simulink model "UNCCModel"  (R2018b)
settings: Solver=ode4  StartTime=0.0  StopTime=Inf  FixedStep=0.025  RelTol=1e-3  EnableMultiTasking=on
PreLoadFcn:
  | preLoadCallback
StartFcn:
  | startCallback
StopFcn:
  | stopCallback
model workspace (MAT data in the model file):
  Ts = 0.025
undefined symbols (not defined in the file or in its folder): acA2000, Ace, Basler, Freerun_FIX_YAW, PoCL
libraries: slrtlib x3, xpcbitflowlib x3, xpcvideoutillib x2, xpcobsoletelib x1, xpcrtudplib x1
(part 2 of 3)

== matlab function UNCCModel/cam3B/Dot_detector_pitch ==
  data: uOut output; u input; roiDims input; locationMethod input; dotConfig input; centroidOverrideCommand input; rCentroidManualOverride input; clusteringParameters input; rCentroidAuto input; r1Img output; r2Img output; rCentroidImg output; viewOptions input
function [uOut,r1Img,r2Img,rCentroidImg] =...
    dotFinder(u,roiDims, locationMethod, dotConfig,centroidOverrideCommand,rCentroidManualOverride,clusteringParameters,rCentroidAuto,viewOptions)
%#codegen
% EXPLANATION OF INPUTS
% u = source image
% roiDims = 4 by 1 vector containing ROI dimensions
% locationMethod = 0 for centroid based dot location
% locationMethod = 1 for cluster based dot location (longer runtime but
% more robust
% dotConfig = 0 for horizontally arranged dots
% dotConfig = 1 for vertically arranged dots
% centroidOverrideCommand = 0 for automatic movemennt of ROI
% centroidOverrideCommand = 1 to use user input as ROI location
% rCentroidManualOverride: 2 element vector where element 1 is x or column
% of ROI centroid and element 2 is y or row of ROI, both of which are
% manually enetered by used
% rCentroidAuto: 2 element vector where element 1 is x or column of ROI
% centroid and element 2 is y or row of ROI, both of which are
% automatically generated from previous iteration
% viewOptions : 8 element vector where each element is a binary on/off
% switch to a certain part of the output view window
%
% WHAT THIS CODE IS
% Method : Centroid Only
% 
% This code is a first attempt at rewriting the code to allow for adaptable
% implemmentation.
% Adaptable implemmentation will ultimately include:
% switch to change between DB clustering and centroid method
% 



%%%%%%%%%%%%%%%%%%%%
% SET ROI DIMENSIONS
%%%%%%%%%%%%%%%%%%%%
[ roiHalfwidth, roiHalfheight ] = getROIDimensions(setToBinary(dotConfig),roiDims); 

%%%%%%%%%%%%%%%%%%%%
% PARSE INPUTS
%%%%%%%%%%%%%%%%%%%%

[dotConfig, locationMethod, centroidOverrideCommand ,rCentroidManualOverride ,viewOptions,roiHalfwidth, roiHalfheight]...
    =parseInputs(dotConfig, locationMethod, centroidOverrideCommand ,rCentroidManualOverride ,viewOptions,roiHalfwidth, roiHalfheight);

%%%%%%%%%%%%%%%%%%%%
%%SET ROI LOCATION%%
%%%%%%%%%%%%%%%%%%%%
rCentroid = rCentroidAuto;
if centroidOverrideCommand == 1  %Override with user input if commanded to do so
    rCentroid = rCentroidManualOverride;
end

%%%%%%%%%%%%%%%%%%%%%%%%%%%%%%%%%%%%
% EXTRACT ROI FROM ORIGIONAL IMAGE %
%%%%%%%%%%%%%%%%%%%%%%%%%%%%%%%%%%%%
roi=u(rCentroid(2) - roiHalfheight : rCentroid(2) + roiHalfheight , rCentroid(1) - roiHalfwidth : rCentroid(1) + roiHalfwidth);

%%%%%%%%%%%%%%%%%%%%%%%%%%%%%
%%%%OTSUS METHOD THRESHOLDING
%%%%%%%%%%%%%%%%%%%%%%%%%%%%%
roi=threshold(roi);


%%%%%%%%%%%%%%%%
% DOT LOCATION %
%%%%%%%%%%%%%%%%
%Preallocate to avoid "Variable undefined on some iteration paths" compile
%error
r1ROI        = [0,0]; r2ROI        = [0,0]; rCentroidROI = [0,0];
if locationMethod == 0; %USE CENTROID BASED METHOD
    if dotConfig == 0 %%HORIZONTAL DOTS
        [r1ROI,r2ROI,rCentroidROI] = centroidMethodHorizontal(roi,roiHalfwidth,roiHalfheight);
    else                %%VERTICAL DOTS
        [r1ROI,r2ROI,rCentroidROI] = centroidMethodVertical(roi,roiHalfwidth,roiHalfheight);
    end
else %USE CLUSTERING BASED METHOD (NOT CURRENTLY IMPLEMENTED)
    %%%REPLACE THIS CODE WITH CLUSTERING METHOD WHEN IMPLEMENTING
    %%%UNCOMMENT CODE BELOW ONCE clusterMethod FUNCTION IS WRITTEN
    %%%[r1ROI,r2ROI,rCentroidROI] = clusterMethod(roi,clusteringParameters);
    if dotConfig == 0 %%HORIZONTAL DOTS
        [r1ROI,r2ROI,rCentroidROI] = centroidMethodHorizontal(roi,roiHalfwidth,roiHalfheight);
    else                %%VERTICAL DOTS
        [r1ROI,r2ROI,rCentroidROI] = centroidMethodVertical(roi,roiHalfwidth,roiHalfheight);
    end
end
%%%%%%%%%%%%%%%%%%%%%%%%%
%%%%PARSE DOT LOCATIONS %
%%%%%%%%%%%%%%%%%%%%%%%%%
%IF DOT CENTER LOCATION ALGORITHM HAS FAILED (OUTPUT = NONSENSE) THEN
%OVERRIDE CENTROID COORDINATES WITH DEFAULT VALUES TO PREVENT PROBLEMS
%LATER
[r1ROI,r2ROI,rCentroidROI] = parseDotLocations(dotConfig,r1ROI,r2ROI,rCentroidROI,roiHalfwidth,roiHalfheight);

%%%%%%%%%%%%%%%%%%%%%%%%%%%%%%%%%%%%%%%%%%%%%%%%%%%
%%%%TRANSFORM BACK TO ORIGIONAL IMAGE COORDINATES %
%%%%%%%%%%%%%%%%%%%%%%%%%%%%%%%%%%%%%%%%%%%%%%%%%%%
%Preallocate to avoid "Variable undefined on some iteration paths" compile
%error
r1Img         = [0,0]; r2Img         = [0,0]; rCenntroidImg = [0,0];

if dotConfig == 0  %HORIZONTALLY ARRANGED DOTS
    [r1Img, r2Img, rCentroidImg] = convertCoordinatesHorizontal(r1ROI,r2ROI,rCentroid,roiHalfwidth,roiHalfheight);
else % VERTICALLY ARRANGED DOTS
    [r1Img, r2Img, rCentroidImg] = convertCoordinatesVertical(r1ROI,r2ROI,rCentroid,roiHalfwidth,roiHalfheight);
end
%%%%%%%%%%%%%%%%%%%%%
% DRAW OUTPUT IMAGE %
%%%%%%%%%%%%%%%%%%%%%

uOut  =  drawOutputImage(viewOptions,u,roi,r1Img,r2Img,rCentroid,r1ROI,r2ROI,roiHalfwidth,roiHalfheight);


end



%DRAW OUTPUT IMAGE
function uOut  =  drawOutputImage(viewOptions,uOut,roi,r1Img,r2Img,rCentroid,r1ROI,r2ROI,roiHalfwidth,roiHalfheight)
%function takes the origional image "u" and redraws it as the output image
%uOut
%View options 7 and 8 are currently not used, can/will be used later for
%clustering algorithm outputs
if viewOptions(1) == 1 %View option = draw any features on output view at all
    if viewOptions(2) == 1 %Draw Features in main image
        if viewOptions(3) == 1 %Draw ROI box in main image
        uOut(rCentroid(2) - roiHalfheight : rCentroid(2) + roiHalfheight, rCentroid(1) - roiHalfwidth                               )=255; %Draw left edge of roi box
        uOut(rCentroid(2) - roiHalfheight : rCentroid(2) + roiHalfheight, rCentroid(1) + roiHalfwidth                               )=255; %Draw right edge of roi box
        uOut(rCentroid(2) - roiHalfheight                               , rCentroid(1) - roiHalfwidth : rCentroid(1)+roiHalfwidth  )=255; %Draw top edge of roi box
        uOut(rCentroid(2) + roiHalfheight                               , rCentroid(1) - roiHalfwidth : rCentroid(1)+roiHalfwidth  )=255; %Draw bottom edge of roi box
        end
        if viewOptions(4) == 1 %Draw crosshairs in main image
            uOut(: ,r1Img(1)  ) = 255;
            uOut(: ,r2Img(1) ) = 255;
            uOut(r1Img(2) ,:  ) = 255;
            uOut(r2Img(2),:  ) = 255;
        end
    end
    if viewOptions(5) == 1 %Draw thresholding in lower left
        roi = 255*roi;
        if viewOptions(6) == 1% Draw crosshairs on thresholding
            roi(r1ROI(2) , :           ) = 255;
            roi(r2ROI(2), :           ) = 255;
            roi(:           , r1ROI(1) ) = 255;
            roi(:           , r2ROI(1)) = 255;
        end
        uOut (1080-size(roi,1)+1:1080, 1:size(roi,2)) = roi;
    end
end
end

%CONVERT ROI COORDINATES TO IMG COORDINATES (HORIZONTAL)
function [rLeftImg, rRightImg, rCentroidImg] = convertCoordinatesHorizontal(rLeftROI,rRightROI,rCentroid,roiHalfwidth,roiHalfheight)
%This function takes in the dot positions in the ROI frame of reference
%and outputs coordinates in the origional image frame of reference, all in
%vectorize format [x,y].  Note that x = column and y = row.

%Convert y (row) coordinates 
yLImg = rCentroid(2) - roiHalfheight + rLeftROI(2);
yRImg = rCentroid(2) - roiHalfheight + rRightROI(2);
%Convert x (col) coordinates
xLImg = rCentroid(1) - roiHalfwidth + rLeftROI(1);
xRImg = rCentroid(1) - roiHalfwidth + rRightROI(1);
%Put results into vector format
rLeftImg  = [ xLImg, yLImg ];
rRightImg = [ xRImg, yRImg ];
%Calculate ROI cenntroid as average of two dot coordinates
rCentroidImg = [fix((xLImg+xRImg)/2),fix((yLImg+yRImg)/2)];

end

%CONVERT ROI COORDINATES TO IMG COORDINATES (VERTICAL)
function [rTopImg, rBottomImg, rCentroidImg] = convertCoordinatesVertical(rTopROI,rBottomROI,rCentroid,roiHalfwidth,roiHalfheight)
%This function takes in the dot positions in the ROI frame of reference
%and outputs coordinates in the origional image frame of reference, all in
%vectorize format [x,y].  Note that x = column and y = row.

%Convert y (row) coordinates 
yTImg = rCentroid(2) - roiHalfheight + rTopROI(2);
yBImg = rCentroid(2) - roiHalfheight + rBottomROI(2);
%Convert x (col) coordinates
xTImg = rCentroid(1) - roiHalfwidth + rTopROI(1);
xBImg = rCentroid(1) - roiHalfwidth + rBottomROI(1);
%Put results into vector format
rTopImg    = [ xTImg, yTImg ];
rBottomImg = [ xBImg, yBImg ];
%Calculate ROI cenntroid as average of two dot coordinates
rCentroidImg = [fix((xTImg+xBImg)/2),fix((yTImg+yBImg)/2)];

end

%CENTROID METHOD DOT LOCATION (HORIZONTAL)
function [rLeft,rRight,rCentroid] = centroidMethodHorizontal(roi,roiHalfwidth,roiHalfheight)
%Function returns the position of the dots rCentroid as well as the
%centroid of the overall image rCentroid
%Calculated by using centroid method, assuming the dots are arranged
%horizontally

%Divide the image in half vertically (left and right)
roiLeft  = roi( : , 1            : roiHalfwidth);
roiRight = roi( : , roiHalfwidth : end         );

%Calculate the x coordinates of the centroids
xLROI = round(sum((sum(roiLeft ,1) .* (1:size(roiLeft ,2))))/sum(sum(roiLeft )));
xRROI = round(sum((sum(roiRight,1) .* (1:size(roiRight,2))))/sum(sum(roiRight)))+roiHalfwidth;
%Calculate the y coordinates of the centroids
yLROI = round(sum((sum(roiLeft ,2) .* (1:size(roiLeft, 1))'))/sum(sum(roiLeft )));
yRROI = round(sum((sum(roiRight,2) .* (1:size(roiRight,1))'))/sum(sum(roiRight)));
%Put results into vector format
rLeft     = [xLROI, yLROI];
rRight    = [xRROI, yRROI];
%Find ROI cenntroid as the average position of the two centroids
rCentroid = [fix((xLROI+xRROI)/2),fix((yLROI+yRROI)/2)];
end

%CENTROID METHOD DOT LOCATION (VERTICAL)
function [rTop,rBottom,rCentroid] = centroidMethodVertical(roi,roiHalfwidth,roiHalfheight)
%Function returns the position of the dots rCentroid as well as the
%centroid of the overall image rCentroid
%Calculated by using centroid method assuming the dots are arranged
%vertically;

%Divide the image in half horizontally (top and bottom)
roiTop    = roi( 1             : roiHalfheight , : );
roiBottom = roi( roiHalfheight : end           , : );

%Calculate the x coordinates of the centroids
xTROI = round(sum((sum(roiTop   ,1) .* (1:size(roiTop   ,2))))/sum(sum(roiTop )));
xBROI = round(sum((sum(roiBottom,1) .* (1:size(roiBottom,2))))/sum(sum(roiBottom)));

%Calculate the y coordinates of the centroids
yTROI = round(sum((sum(roiTop   ,2) .* (1:size(roiTop   ,1))'))/sum(sum(roiTop )));
yBROI = round(sum((sum(roiBottom,2) .* (1:size(roiBottom,1))'))/sum(sum(roiBottom)))+roiHalfheight;
%Put results into vector format
rTop     = [xTROI, yTROI];
rBottom  = [xBROI, yBROI];
%Find ROI cenntroid as the average position of the two centroids
rCentroid = [fix((xTROI+xBROI)/2),fix((yTROI+yBROI)/2)];
end

%CLUSTERING METHOD DOT LOCATION
function [rTop,rBottom,rCentroid] = clusterMethod(roi,clusteringParameters)
%This function is currently a placeholder, will be used later if/when
%clustering is implemented
end

%IMAGE THRESHOLDING - OTSU'S METHOD
function img = threshold(img)
%This function takes in a grayscale matrix and outputs a thresholded,
%binaray matrix according to Otsus Method.

%Generate histogram of image
counts=zeros(256,1);
[m,n]=size(img);
for i = 1:m*n
    counts(img(i)+1)=counts(img(i)+1)+1;
end
%Callculate variances
p = counts / sum(counts);
sigma_b=zeros(256,1);
%%%%%%%%%%%%%%%%55
%POSSIBLE DIV BY ZERO ERRORS HERE?
%%%%%%%%%%%%%%%%%%%%%%
for t = 1 : 256
    q_L = sum(p(1 : t));
    q_H = sum(p(t + 1 : end));
    miu_L = sum(p(1 : t) .* (1 : t)') / q_L;
    miu_H = sum(p(t + 1 : end) .* (t + 1 : 256)') / q_H;
    sigma_b(t) = q_L * q_H * (miu_L - miu_H)^2;
end
% Desired threshold is the max of sigma_b vector
[~,threshold_otsu] = max(sigma_b(:));
% Threshold image as those points above the threshold value
img=(img>threshold_otsu);
end

%INPUT PARSING
function        [dotConfig, locationMethod, centroidOverrideCommand ,rCentroidManualOverride ,viewOptions,roiHalfwidth, roiHalfheight]...
    =parseInputs(dotConfig, locationMethod, centroidOverrideCommand ,rCentroidManualOverride ,viewOptions,roiHalfwidth, roiHalfheight)
% This function parses inputs and corrects potentially harmful/unstable
% inputs.  
locationMethod            = setToBinary(locationMethod);
centroidOverrideCommand   = setToBinary(centroidOverrideCommand);

if centroidOverrideCommand == 1
    if numel(rCentroidManualOverride)~=2
        rCentroidManualOverride = [540,1020];
    end
    if rCentroidManualOverride(2) > 1080 - roiHalfheight - 1
        rCentroidManualOverride(2) = 1080 - roiHalfheight - 1;
    end
    if rCentroidManualOverride(1) > 2040 - roiHalfwidth - 1
        rCentroidManualOverride(1) = 2040 - roiHalfwidth - 1;
    end
    
    if rCentroidManualOverride(2) < roiHalfheight + 1
        rCentroidManualOverride(2) = roiHalfheight + 1;
    end
    if rCentroidManualOverride(1) < roiHalfwidth + 1
        rCentroidManualOverride(1) = roiHalfwidth + 1;
    end
    
    
end

if numel(viewOptions) > 8
    viewOptions = viewOptions(1:8);
end
if numel(viewOptions) < 8
    viewOptions = [0,0,0,0,0,0,0,0];
end
for i=1:8
    viewOptions(i) = setToBinary(viewOptions(i));
end
rCentroidManualOverride=fix(rCentroidManualOverride);
dotConfig = setToBinary(dotConfig);

end

%ROUND TO BINARY VALUE
function [out] = setToBinary(in)
%takes any numerical input and sets it to either 0 or 1 depending on
%what's closer
out = in;
if out>1
    out=1;
end
if out<0
    out=0;
end
if out >0  && out <1
    out=round(out);
end
end

%GET ROI DIMENSIONS
function [roiHalfwidth,roiHalfheight] = getROIDimensions(dotConfig,roiDims)
%This function sets the ROI Dimensions depending on user input
%(dotConfig).


if numel(roiDims)==4 %Check to make sure ROI dimension vector is right length
    for i = 1 : 4   %Saturation, make sure roi dimension vector elements make sense, if not set them to something more reasonable
       if roiDims(i)>200
           roiDims(i)=200;
       end
       
       if roiDims(i)<20
           roiDims(i)=20;
       end
    end
    
    
    
    if dotConfig == 1 %VERTICAL ARRANGEMENT
        roiHalfwidth = roiDims(1);
        roiHalfheight = roiDims(2);
        
    else
        roiHalfwidth = roiDims(3);
        roiHalfheight = roiDims(4);
    end
end

end

%PARSE DOT LOCATIONS
function [r1ROI,r2ROI,rCentroidROI] = parseDotLocations(dotConfig,r1ROI,r2ROI,rCentroidROI,roiHalfwidth,roiHalfheight)
if dotConfig == 0 %HORIZONTAL DOTS
    if isnan(r1ROI(1))
        r1ROI(1)=fix(roiHalfwidth/2);
    end
    if isnan(r1ROI(2))
        r1ROI(2)=roiHalfheight;
    end
    if isnan(r2ROI(1))
        r2ROI(1)=fix(3*roiHalfheight/2);
    end
    if isnan(r2ROI(2))
        r2ROI(2)=roiHalfheight;
    end
else %VERTICAL DOTS
    if isnan(r1ROI(1))
        r1ROI(1)=roiHalfwidth;
    end
    if isnan(r1ROI(2))
        r1ROI(2)=fix(roiHalfheight/2);
    end
    if isnan(r2ROI(1))
        r2ROI(1)=roiHalfwidth;
    end
    if isnan(r2ROI(2))
        r2ROI(2)=fix(3*roiHalfheight/2);
    end
end

if isnan(rCentroidROI(1))
   rCentroidROI(1)=roiHalfwidth;
end

if isnan(rCentroidROI(2))
    rCentroidROI(2) = roiHalfheight;
end


end

== matlab function UNCCModel/findPositions1 ==
  data: R input; rSideGF output; rBottomAGF output; rCOM input; rBottomBGF output; rSideBF input; rBottomABF input; rBottomBBF input
function [rSideGF,rBottomAGF,rBottomBGF] = ...
    findDotPositions(R,rCOM,rSideBF,rBottomABF,rBottomBBF)
%#codegen

rSideGF    = rCOM + R*rSideBF;
rBottomAGF = rCOM + R*rBottomABF;
rBottomBGF = rCOM + R*rBottomABF;

== matlab function UNCCModel/findPositions ==
  data: x1 output; x2 output; rSideGF input; y1 output; y2 output; rBottomAGF input; rBottomBGF input; R input; rSideBF input; rBottomABF input; rBottomBBF input; z output
function [x1,x2,y1,y2,z] = ...
    findPositions(rSideGF,rBottomAGF,rBottomBGF,R,rSideBF,rBottomABF,rBottomBBF)
%#codegen

% Find x from side camera
% Find y from bottom A dots
x1 = rBottomAGF(1);
y1 = rBottomAGF(2);

x1 = x1 - (R(1,1)*rSideBF(1)    + R(1,2)*rSideBF(2)    + R(1,3)*rSideBF(3));
y1 = y1 - (R(2,1)*rBottomABF(1) + R(2,2)*rBottomABF(2) + R(2,3)*rBottomABF(3));

% Find x from bottom A dots
% Find y from bottom B dots
% Note: these values are not used in the model, just logged.
x2 = rSideGF(1);
y2 = rBottomBGF(2);

x2 = x2 - (R(1,1)*rBottomABF(1) + R(1,2)*rBottomABF(2) + R(1,3)*rBottomABF(3));
y2 = y2 - (R(2,1)*rBottomBBF(1) + R(2,2)*rBottomBBF(2) + R(2,3)*rBottomBBF(3));

% Find z from side camera (only way possible).
z = rSideGF(3);
z = z - (R(3,1)*rSideBF(1)    + R(3,2)*rSideBF(2)    + R(3,3)*rSideBF(3));

== matlab function UNCCModel/cam2/Dot_detector_pitch ==
  data: uOut output; u input; roiDims input; locationMethod input; dotConfig input; centroidOverrideCommand input; rCentroidManualOverride input; clusteringParameters input; rCentroidAuto input; r1Img output; r2Img output; rCentroidImg output; viewOptions input
function [uOut,r1Img,r2Img,rCentroidImg] =...
    dotFinder(u,roiDims, locationMethod, dotConfig,centroidOverrideCommand,rCentroidManualOverride,clusteringParameters,rCentroidAuto,viewOptions)
%#codegen
% EXPLANATION OF INPUTS
% u = source image
% roiDims = 4 by 1 vector containing ROI dimensions
% locationMethod = 0 for centroid based dot location
% locationMethod = 1 for cluster based dot location (longer runtime but
% more robust
% dotConfig = 0 for horizontally arranged dots
% dotConfig = 1 for vertically arranged dots
% centroidOverrideCommand = 0 for automatic movemennt of ROI
% centroidOverrideCommand = 1 to use user input as ROI location
% rCentroidManualOverride: 2 element vector where element 1 is x or column
% of ROI centroid and element 2 is y or row of ROI, both of which are
% manually enetered by used
% rCentroidAuto: 2 element vector where element 1 is x or column of ROI
% centroid and element 2 is y or row of ROI, both of which are
% automatically generated from previous iteration
% viewOptions : 8 element vector where each element is a binary on/off
% switch to a certain part of the output view window
%
% WHAT THIS CODE IS
% Method : Centroid Only
% 
% This code is a first attempt at rewriting the code to allow for adaptable
% implemmentation.
% Adaptable implemmentation will ultimately include:
% switch to change between DB clustering and centroid method
% 



%%%%%%%%%%%%%%%%%%%%
% SET ROI DIMENSIONS
%%%%%%%%%%%%%%%%%%%%
[ roiHalfwidth, roiHalfheight ] = getROIDimensions(setToBinary(dotConfig),roiDims); 

%%%%%%%%%%%%%%%%%%%%
% PARSE INPUTS
%%%%%%%%%%%%%%%%%%%%

[dotConfig, locationMethod, centroidOverrideCommand ,rCentroidManualOverride ,viewOptions,roiHalfwidth, roiHalfheight]...
    =parseInputs(dotConfig, locationMethod, centroidOverrideCommand ,rCentroidManualOverride ,viewOptions,roiHalfwidth, roiHalfheight);

%%%%%%%%%%%%%%%%%%%%
%%SET ROI LOCATION%%
%%%%%%%%%%%%%%%%%%%%
rCentroid = rCentroidAuto;
if centroidOverrideCommand == 1  %Override with user input if commanded to do so
    rCentroid = rCentroidManualOverride;
end

%%%%%%%%%%%%%%%%%%%%%%%%%%%%%%%%%%%%
% EXTRACT ROI FROM ORIGIONAL IMAGE %
%%%%%%%%%%%%%%%%%%%%%%%%%%%%%%%%%%%%
roi=u(rCentroid(2) - roiHalfheight : rCentroid(2) + roiHalfheight , rCentroid(1) - roiHalfwidth : rCentroid(1) + roiHalfwidth);

%%%%%%%%%%%%%%%%%%%%%%%%%%%%%
%%%%OTSUS METHOD THRESHOLDING
%%%%%%%%%%%%%%%%%%%%%%%%%%%%%
roi=threshold(roi);


%%%%%%%%%%%%%%%%
% DOT LOCATION %
%%%%%%%%%%%%%%%%
%Preallocate to avoid "Variable undefined on some iteration paths" compile
%error
r1ROI        = [0,0]; r2ROI        = [0,0]; rCentroidROI = [0,0];
if locationMethod == 0; %USE CENTROID BASED METHOD
    if dotConfig == 0 %%HORIZONTAL DOTS
        [r1ROI,r2ROI,rCentroidROI] = centroidMethodHorizontal(roi,roiHalfwidth,roiHalfheight);
    else                %%VERTICAL DOTS
        [r1ROI,r2ROI,rCentroidROI] = centroidMethodVertical(roi,roiHalfwidth,roiHalfheight);
    end
else %USE CLUSTERING BASED METHOD (NOT CURRENTLY IMPLEMENTED)
    %%%REPLACE THIS CODE WITH CLUSTERING METHOD WHEN IMPLEMENTING
    %%%UNCOMMENT CODE BELOW ONCE clusterMethod FUNCTION IS WRITTEN
    %%%[r1ROI,r2ROI,rCentroidROI] = clusterMethod(roi,clusteringParameters);
    if dotConfig == 0 %%HORIZONTAL DOTS
        [r1ROI,r2ROI,rCentroidROI] = centroidMethodHorizontal(roi,roiHalfwidth,roiHalfheight);
    else                %%VERTICAL DOTS
        [r1ROI,r2ROI,rCentroidROI] = centroidMethodVertical(roi,roiHalfwidth,roiHalfheight);
    end
end
%%%%%%%%%%%%%%%%%%%%%%%%%
%%%%PARSE DOT LOCATIONS %
%%%%%%%%%%%%%%%%%%%%%%%%%
%IF DOT CENTER LOCATION ALGORITHM HAS FAILED (OUTPUT = NONSENSE) THEN
%OVERRIDE CENTROID COORDINATES WITH DEFAULT VALUES TO PREVENT PROBLEMS
%LATER
[r1ROI,r2ROI,rCentroidROI] = parseDotLocations(dotConfig,r1ROI,r2ROI,rCentroidROI,roiHalfwidth,roiHalfheight);

%%%%%%%%%%%%%%%%%%%%%%%%%%%%%%%%%%%%%%%%%%%%%%%%%%%
%%%%TRANSFORM BACK TO ORIGIONAL IMAGE COORDINATES %
%%%%%%%%%%%%%%%%%%%%%%%%%%%%%%%%%%%%%%%%%%%%%%%%%%%
%Preallocate to avoid "Variable undefined on some iteration paths" compile
%error
r1Img         = [0,0]; r2Img         = [0,0]; rCenntroidImg = [0,0];

if dotConfig == 0  %HORIZONTALLY ARRANGED DOTS
    [r1Img, r2Img, rCentroidImg] = convertCoordinatesHorizontal(r1ROI,r2ROI,rCentroid,roiHalfwidth,roiHalfheight);
else % VERTICALLY ARRANGED DOTS
    [r1Img, r2Img, rCentroidImg] = convertCoordinatesVertical(r1ROI,r2ROI,rCentroid,roiHalfwidth,roiHalfheight);
end
%%%%%%%%%%%%%%%%%%%%%
% DRAW OUTPUT IMAGE %
%%%%%%%%%%%%%%%%%%%%%

uOut  =  drawOutputImage(viewOptions,u,roi,r1Img,r2Img,rCentroid,r1ROI,r2ROI,roiHalfwidth,roiHalfheight);


end



%DRAW OUTPUT IMAGE
function uOut  =  drawOutputImage(viewOptions,uOut,roi,r1Img,r2Img,rCentroid,r1ROI,r2ROI,roiHalfwidth,roiHalfheight)
%function takes the origional image "u" and redraws it as the output image
%uOut
%View options 7 and 8 are currently not used, can/will be used later for
%clustering algorithm outputs
if viewOptions(1) == 1 %View option = draw any features on output view at all
    if viewOptions(2) == 1 %Draw Features in main image
        if viewOptions(3) == 1 %Draw ROI box in main image
        uOut(rCentroid(2) - roiHalfheight : rCentroid(2) + roiHalfheight, rCentroid(1) - roiHalfwidth                               )=255; %Draw left edge of roi box
        uOut(rCentroid(2) - roiHalfheight : rCentroid(2) + roiHalfheight, rCentroid(1) + roiHalfwidth                               )=255; %Draw right edge of roi box
        uOut(rCentroid(2) - roiHalfheight                               , rCentroid(1) - roiHalfwidth : rCentroid(1)+roiHalfwidth  )=255; %Draw top edge of roi box
        uOut(rCentroid(2) + roiHalfheight                               , rCentroid(1) - roiHalfwidth : rCentroid(1)+roiHalfwidth  )=255; %Draw bottom edge of roi box
        end
        if viewOptions(4) == 1 %Draw crosshairs in main image
            uOut(: ,r1Img(1)  ) = 255;
            uOut(: ,r2Img(1) ) = 255;
            uOut(r1Img(2) ,:  ) = 255;
            uOut(r2Img(2),:  ) = 255;
        end
    end
    if viewOptions(5) == 1 %Draw thresholding in lower left
        roi = 255*roi;
        if viewOptions(6) == 1% Draw crosshairs on thresholding
            roi(r1ROI(2) , :           ) = 255;
            roi(r2ROI(2), :           ) = 255;
            roi(:           , r1ROI(1) ) = 255;
            roi(:           , r2ROI(1)) = 255;
        end
        uOut (1080-size(roi,1)+1:1080, 1:size(roi,2)) = roi;
    end
end
end

%CONVERT ROI COORDINATES TO IMG COORDINATES (HORIZONTAL)
function [rLeftImg, rRightImg, rCentroidImg] = convertCoordinatesHorizontal(rLeftROI,rRightROI,rCentroid,roiHalfwidth,roiHalfheight)
%This function takes in the dot positions in the ROI frame of reference
%and outputs coordinates in the origional image frame of reference, all in
%vectorize format [x,y].  Note that x = column and y = row.

%Convert y (row) coordinates 
yLImg = rCentroid(2) - roiHalfheight + rLeftROI(2);
yRImg = rCentroid(2) - roiHalfheight + rRightROI(2);
%Convert x (col) coordinates
xLImg = rCentroid(1) - roiHalfwidth + rLeftROI(1);
xRImg = rCentroid(1) - roiHalfwidth + rRightROI(1);
%Put results into vector format
rLeftImg  = [ xLImg, yLImg ];
rRightImg = [ xRImg, yRImg ];
%Calculate ROI cenntroid as average of two dot coordinates
rCentroidImg = [fix((xLImg+xRImg)/2),fix((yLImg+yRImg)/2)];

end

%CONVERT ROI COORDINATES TO IMG COORDINATES (VERTICAL)
function [rTopImg, rBottomImg, rCentroidImg] = convertCoordinatesVertical(rTopROI,rBottomROI,rCentroid,roiHalfwidth,roiHalfheight)
%This function takes in the dot positions in the ROI frame of reference
%and outputs coordinates in the origional image frame of reference, all in
%vectorize format [x,y].  Note that x = column and y = row.

%Convert y (row) coordinates 
yTImg = rCentroid(2) - roiHalfheight + rTopROI(2);
yBImg = rCentroid(2) - roiHalfheight + rBottomROI(2);
%Convert x (col) coordinates
xTImg = rCentroid(1) - roiHalfwidth + rTopROI(1);
xBImg = rCentroid(1) - roiHalfwidth + rBottomROI(1);
%Put results into vector format
rTopImg    = [ xTImg, yTImg ];
rBottomImg = [ xBImg, yBImg ];
%Calculate ROI cenntroid as average of two dot coordinates
rCentroidImg = [fix((xTImg+xBImg)/2),fix((yTImg+yBImg)/2)];

end

%CENTROID METHOD DOT LOCATION (HORIZONTAL)
function [rLeft,rRight,rCentroid] = centroidMethodHorizontal(roi,roiHalfwidth,roiHalfheight)
%Function returns the position of the dots rCentroid as well as the
%centroid of the overall image rCentroid
%Calculated by using centroid method, assuming the dots are arranged
%horizontally

%Divide the image in half vertically (left and right)
roiLeft  = roi( : , 1            : roiHalfwidth);
roiRight = roi( : , roiHalfwidth : end         );

%Calculate the x coordinates of the centroids
xLROI = round(sum((sum(roiLeft ,1) .* (1:size(roiLeft ,2))))/sum(sum(roiLeft )));
xRROI = round(sum((sum(roiRight,1) .* (1:size(roiRight,2))))/sum(sum(roiRight)))+roiHalfwidth;
%Calculate the y coordinates of the centroids
yLROI = round(sum((sum(roiLeft ,2) .* (1:size(roiLeft, 1))'))/sum(sum(roiLeft )));
yRROI = round(sum((sum(roiRight,2) .* (1:size(roiRight,1))'))/sum(sum(roiRight)));
%Put results into vector format
rLeft     = [xLROI, yLROI];
rRight    = [xRROI, yRROI];
%Find ROI cenntroid as the average position of the two centroids
rCentroid = [fix((xLROI+xRROI)/2),fix((yLROI+yRROI)/2)];
end

%CENTROID METHOD DOT LOCATION (VERTICAL)
function [rTop,rBottom,rCentroid] = centroidMethodVertical(roi,roiHalfwidth,roiHalfheight)
%Function returns the position of the dots rCentroid as well as the
%centroid of the overall image rCentroid
%Calculated by using centroid method assuming the dots are arranged
%vertically;

%Divide the image in half horizontally (top and bottom)
roiTop    = roi( 1             : roiHalfheight , : );
roiBottom = roi( roiHalfheight : end           , : );

%Calculate the x coordinates of the centroids
xTROI = round(sum((sum(roiTop   ,1) .* (1:size(roiTop   ,2))))/sum(sum(roiTop )));
xBROI = round(sum((sum(roiBottom,1) .* (1:size(roiBottom,2))))/sum(sum(roiBottom)));

%Calculate the y coordinates of the centroids
yTROI = round(sum((sum(roiTop   ,2) .* (1:size(roiTop   ,1))'))/sum(sum(roiTop )));
yBROI = round(sum((sum(roiBottom,2) .* (1:size(roiBottom,1))'))/sum(sum(roiBottom)))+roiHalfheight;
%Put results into vector format
rTop     = [xTROI, yTROI];
rBottom  = [xBROI, yBROI];
%Find ROI cenntroid as the average position of the two centroids
rCentroid = [fix((xTROI+xBROI)/2),fix((yTROI+yBROI)/2)];
end

%CLUSTERING METHOD DOT LOCATION
function [rTop,rBottom,rCentroid] = clusterMethod(roi,clusteringParameters)
%This function is currently a placeholder, will be used later if/when
%clustering is implemented
end

%IMAGE THRESHOLDING - OTSU'S METHOD
function img = threshold(img)
%This function takes in a grayscale matrix and outputs a thresholded,
%binaray matrix according to Otsus Method.

%Generate histogram of image
counts=zeros(256,1);
[m,n]=size(img);
for i = 1:m*n
    counts(img(i)+1)=counts(img(i)+1)+1;
end
%Callculate variances
p = counts / sum(counts);
sigma_b=zeros(256,1);
%%%%%%%%%%%%%%%%55
%POSSIBLE DIV BY ZERO ERRORS HERE?
%%%%%%%%%%%%%%%%%%%%%%
for t = 1 : 256
    q_L = sum(p(1 : t));
    q_H = sum(p(t + 1 : end));
    miu_L = sum(p(1 : t) .* (1 : t)') / q_L;
    miu_H = sum(p(t + 1 : end) .* (t + 1 : 256)') / q_H;
    sigma_b(t) = q_L * q_H * (miu_L - miu_H)^2;
end
% Desired threshold is the max of sigma_b vector
[~,threshold_otsu] = max(sigma_b(:));
% Threshold image as those points above the threshold value
img=(img>threshold_otsu);
end

%INPUT PARSING
function        [dotConfig, locationMethod, centroidOverrideCommand ,rCentroidManualOverride ,viewOptions,roiHalfwidth, roiHalfheight]...
    =parseInputs(dotConfig, locationMethod, centroidOverrideCommand ,rCentroidManualOverride ,viewOptions,roiHalfwidth, roiHalfheight)
% This function parses inputs and corrects potentially harmful/unstable
% inputs.  
locationMethod            = setToBinary(locationMethod);
centroidOverrideCommand   = setToBinary(centroidOverrideCommand);

if centroidOverrideCommand == 1
    if numel(rCentroidManualOverride)~=2
        rCentroidManualOverride = [540,1020];
    end
    if rCentroidManualOverride(2) > 1080 - roiHalfheight - 1
        rCentroidManualOverride(2) = 1080 - roiHalfheight - 1;
    end
    if rCentroidManualOverride(1) > 2040 - roiHalfwidth - 1
        rCentroidManualOverride(1) = 2040 - roiHalfwidth - 1;
    end
    
    if rCentroidManualOverride(2) < roiHalfheight + 1
        rCentroidManualOverride(2) = roiHalfheight + 1;
    end
    if rCentroidManualOverride(1) < roiHalfwidth + 1
        rCentroidManualOverride(1) = roiHalfwidth + 1;
    end
    
    
end

if numel(viewOptions) > 8
    viewOptions = viewOptions(1:8);
end
if numel(viewOptions) < 8
    viewOptions = [0,0,0,0,0,0,0,0];
end
for i=1:8
    viewOptions(i) = setToBinary(viewOptions(i));
end
rCentroidManualOverride=fix(rCentroidManualOverride);
dotConfig = setToBinary(dotConfig);

end

%ROUND TO BINARY VALUE
function [out] = setToBinary(in)
%takes any numerical input and sets it to either 0 or 1 depending on
%what's closer
out = in;
if out>1
    out=1;
end
if out<0
    out=0;
end
if out >0  && out <1
    out=round(out);
end
end

%GET ROI DIMENSIONS
function [roiHalfwidth,roiHalfheight] = getROIDimensions(dotConfig,roiDims)
%This function sets the ROI Dimensions depending on user input
%(dotConfig).


if numel(roiDims)==4 %Check to make sure ROI dimension vector is right length
    for i = 1 : 4   %Saturation, make sure roi dimension vector elements make sense, if not set them to something more reasonable
       if roiDims(i)>500
           roiDims(i)=500;
       end
       
       if roiDims(i)<20
           roiDims(i)=20;
       end
    end
    
    
    
    if dotConfig == 1 %VERTICAL ARRANGEMENT
        roiHalfwidth = roiDims(1);
        roiHalfheight = roiDims(2);
        
    else
        roiHalfwidth = roiDims(3);
        roiHalfheight = roiDims(4);
    end
end

end

%PARSE DOT LOCATIONS
function [r1ROI,r2ROI,rCentroidROI] = parseDotLocations(dotConfig,r1ROI,r2ROI,rCentroidROI,roiHalfwidth,roiHalfheight)
if dotConfig == 0 %HORIZONTAL DOTS
    if isnan(r1ROI(1))
        r1ROI(1)=fix(roiHalfwidth/2);
    end
    if isnan(r1ROI(2))
        r1ROI(2)=roiHalfheight;
    end
    if isnan(r2ROI(1))
        r2ROI(1)=fix(3*roiHalfheight/2);
    end
    if isnan(r2ROI(2))
        r2ROI(2)=roiHalfheight;
    end
else %VERTICAL DOTS
    if isnan(r1ROI(1))
        r1ROI(1)=roiHalfwidth;
    end
    if isnan(r1ROI(2))
        r1ROI(2)=fix(roiHalfheight/2);
    end
    if isnan(r2ROI(1))
        r2ROI(1)=roiHalfwidth;
    end
    if isnan(r2ROI(2))
        r2ROI(2)=fix(3*roiHalfheight/2);
    end
end

if isnan(rCentroidROI(1))
   rCentroidROI(1)=roiHalfwidth;
end

if isnan(rCentroidROI(2))
    rCentroidROI(2) = roiHalfheight;
end


end

== matlab function UNCCModel/rollSetpointGeneration ==
  data: signalType input; time input; setPoint output; amp input; freq input
function setPoint  = fcn(signalType,time, amp, freq)
%#codegen
setPoint = amp*sin(2*pi*freq*time);
if signalType == 2
setPoint = amp*sign(setPoint);
end
end

== matlab function UNCCModel/cam3A/Dot_detector_pitch ==
  data: uOut output; u input; roiDims input; locationMethod input; dotConfig input; centroidOverrideCommand input; rCentroidManualOverride input; clusteringParameters input; rCentroidAuto input; r1Img output; r2Img output; rCentroidImg output; viewOptions input
function [uOut,r1Img,r2Img,rCentroidImg] =...
    dotFinder(u,roiDims, locationMethod, dotConfig,centroidOverrideCommand,rCentroidManualOverride,clusteringParameters,rCentroidAuto,viewOptions)
%#codegen
% EXPLANATION OF INPUTS
% u = source image
% roiDims = 4 by 1 vector containing ROI dimensions
% locationMethod = 0 for centroid based dot location
% locationMethod = 1 for cluster based dot location (longer runtime but
% more robust
% dotConfig = 0 for horizontally arranged dots
% dotConfig = 1 for vertically arranged dots
% centroidOverrideCommand = 0 for automatic movemennt of ROI
% centroidOverrideCommand = 1 to use user input as ROI location
% rCentroidManualOverride: 2 element vector where element 1 is x or column
% of ROI centroid and element 2 is y or row of ROI, both of which are
% manually enetered by used
% rCentroidAuto: 2 element vector where element 1 is x or column of ROI
% centroid and element 2 is y or row of ROI, both of which are
% automatically generated from previous iteration
% viewOptions : 8 element vector where each element is a binary on/off
% switch to a certain part of the output view window
%
% WHAT THIS CODE IS
% Method : Centroid Only
% 
% This code is a first attempt at rewriting the code to allow for adaptable
% implemmentation.
% Adaptable implemmentation will ultimately include:
% switch to change between DB clustering and centroid method
% 



%%%%%%%%%%%%%%%%%%%%
% SET ROI DIMENSIONS
%%%%%%%%%%%%%%%%%%%%
[ roiHalfwidth, roiHalfheight ] = getROIDimensions(setToBinary(dotConfig),roiDims); 

%%%%%%%%%%%%%%%%%%%%
% PARSE INPUTS
%%%%%%%%%%%%%%%%%%%%

[dotConfig, locationMethod, centroidOverrideCommand ,rCentroidManualOverride ,viewOptions,roiHalfwidth, roiHalfheight]...
    =parseInputs(dotConfig, locationMethod, centroidOverrideCommand ,rCentroidManualOverride ,viewOptions,roiHalfwidth, roiHalfheight);

%%%%%%%%%%%%%%%%%%%%
%%SET ROI LOCATION%%
%%%%%%%%%%%%%%%%%%%%
rCentroid = rCentroidAuto;
if centroidOverrideCommand == 1  %Override with user input if commanded to do so
    rCentroid = rCentroidManualOverride;
end

%%%%%%%%%%%%%%%%%%%%%%%%%%%%%%%%%%%%
% EXTRACT ROI FROM ORIGIONAL IMAGE %
%%%%%%%%%%%%%%%%%%%%%%%%%%%%%%%%%%%%
roi=u(rCentroid(2) - roiHalfheight : rCentroid(2) + roiHalfheight , rCentroid(1) - roiHalfwidth : rCentroid(1) + roiHalfwidth);

%%%%%%%%%%%%%%%%%%%%%%%%%%%%%
%%%%OTSUS METHOD THRESHOLDING
%%%%%%%%%%%%%%%%%%%%%%%%%%%%%
roi=threshold(roi);


%%%%%%%%%%%%%%%%
% DOT LOCATION %
%%%%%%%%%%%%%%%%
%Preallocate to avoid "Variable undefined on some iteration paths" compile
%error
r1ROI        = [0,0]; r2ROI        = [0,0]; rCentroidROI = [0,0];
if locationMethod == 0; %USE CENTROID BASED METHOD
    if dotConfig == 0 %%HORIZONTAL DOTS
        [r1ROI,r2ROI,rCentroidROI] = centroidMethodHorizontal(roi,roiHalfwidth,roiHalfheight);
    else                %%VERTICAL DOTS
        [r1ROI,r2ROI,rCentroidROI] = centroidMethodVertical(roi,roiHalfwidth,roiHalfheight);
    end
else %USE CLUSTERING BASED METHOD (NOT CURRENTLY IMPLEMENTED)
    %%%REPLACE THIS CODE WITH CLUSTERING METHOD WHEN IMPLEMENTING
    %%%UNCOMMENT CODE BELOW ONCE clusterMethod FUNCTION IS WRITTEN
    %%%[r1ROI,r2ROI,rCentroidROI] = clusterMethod(roi,clusteringParameters);
    if dotConfig == 0 %%HORIZONTAL DOTS
        [r1ROI,r2ROI,rCentroidROI] = centroidMethodHorizontal(roi,roiHalfwidth,roiHalfheight);
    else                %%VERTICAL DOTS
        [r1ROI,r2ROI,rCentroidROI] = centroidMethodVertical(roi,roiHalfwidth,roiHalfheight);
    end
end
%%%%%%%%%%%%%%%%%%%%%%%%%
%%%%PARSE DOT LOCATIONS %
%%%%%%%%%%%%%%%%%%%%%%%%%
%IF DOT CENTER LOCATION ALGORITHM HAS FAILED (OUTPUT = NONSENSE) THEN
%OVERRIDE CENTROID COORDINATES WITH DEFAULT VALUES TO PREVENT PROBLEMS
%LATER
[r1ROI,r2ROI,rCentroidROI] = parseDotLocations(dotConfig,r1ROI,r2ROI,rCentroidROI,roiHalfwidth,roiHalfheight);

%%%%%%%%%%%%%%%%%%%%%%%%%%%%%%%%%%%%%%%%%%%%%%%%%%%
%%%%TRANSFORM BACK TO ORIGIONAL IMAGE COORDINATES %
%%%%%%%%%%%%%%%%%%%%%%%%%%%%%%%%%%%%%%%%%%%%%%%%%%%
%Preallocate to avoid "Variable undefined on some iteration paths" compile
%error
r1Img         = [0,0]; r2Img         = [0,0]; rCenntroidImg = [0,0];

if dotConfig == 0  %HORIZONTALLY ARRANGED DOTS
    [r1Img, r2Img, rCentroidImg] = convertCoordinatesHorizontal(r1ROI,r2ROI,rCentroid,roiHalfwidth,roiHalfheight);
else % VERTICALLY ARRANGED DOTS
    [r1Img, r2Img, rCentroidImg] = convertCoordinatesVertical(r1ROI,r2ROI,rCentroid,roiHalfwidth,roiHalfheight);
end
%%%%%%%%%%%%%%%%%%%%%
% DRAW OUTPUT IMAGE %
%%%%%%%%%%%%%%%%%%%%%

uOut  =  drawOutputImage(viewOptions,u,roi,r1Img,r2Img,rCentroid,r1ROI,r2ROI,roiHalfwidth,roiHalfheight);


end



%DRAW OUTPUT IMAGE
function uOut  =  drawOutputImage(viewOptions,uOut,roi,r1Img,r2Img,rCentroid,r1ROI,r2ROI,roiHalfwidth,roiHalfheight)
%function takes the origional image "u" and redraws it as the output image
%uOut
%View options 7 and 8 are currently not used, can/will be used later for
%clustering algorithm outputs
if viewOptions(1) == 1 %View option = draw any features on output view at all
    if viewOptions(2) == 1 %Draw Features in main image
        if viewOptions(3) == 1 %Draw ROI box in main image
        uOut(rCentroid(2) - roiHalfheight : rCentroid(2) + roiHalfheight, rCentroid(1) - roiHalfwidth                               )=255; %Draw left edge of roi box
        uOut(rCentroid(2) - roiHalfheight : rCentroid(2) + roiHalfheight, rCentroid(1) + roiHalfwidth                               )=255; %Draw right edge of roi box
        uOut(rCentroid(2) - roiHalfheight                               , rCentroid(1) - roiHalfwidth : rCentroid(1)+roiHalfwidth  )=255; %Draw top edge of roi box
        uOut(rCentroid(2) + roiHalfheight                               , rCentroid(1) - roiHalfwidth : rCentroid(1)+roiHalfwidth  )=255; %Draw bottom edge of roi box
        end
        if viewOptions(4) == 1 %Draw crosshairs in main image
            uOut(: ,r1Img(1)  ) = 255;
            uOut(: ,r2Img(1) ) = 255;
            uOut(r1Img(2) ,:  ) = 255;
            uOut(r2Img(2),:  ) = 255;
        end
    end
    if viewOptions(5) == 1 %Draw thresholding in lower left
        roi = 255*roi;
        if viewOptions(6) == 1% Draw crosshairs on thresholding
            roi(r1ROI(2) , :           ) = 255;
            roi(r2ROI(2), :           ) = 255;
            roi(:           , r1ROI(1) ) = 255;
            roi(:           , r2ROI(1)) = 255;
        end
        uOut (1080-size(roi,1)+1:1080, 1:size(roi,2)) = roi;
    end
end
end

%CONVERT ROI COORDINATES TO IMG COORDINATES (HORIZONTAL)
function [rLeftImg, rRightImg, rCentroidImg] = convertCoordinatesHorizontal(rLeftROI,rRightROI,rCentroid,roiHalfwidth,roiHalfheight)
%This function takes in the dot positions in the ROI frame of reference
%and outputs coordinates in the origional image frame of reference, all in
%vectorize format [x,y].  Note that x = column and y = row.

%Convert y (row) coordinates 
yLImg = rCentroid(2) - roiHalfheight + rLeftROI(2);
yRImg = rCentroid(2) - roiHalfheight + rRightROI(2);
%Convert x (col) coordinates
xLImg = rCentroid(1) - roiHalfwidth + rLeftROI(1);
xRImg = rCentroid(1) - roiHalfwidth + rRightROI(1);
%Put results into vector format
rLeftImg  = [ xLImg, yLImg ];
rRightImg = [ xRImg, yRImg ];
%Calculate ROI cenntroid as average of two dot coordinates
rCentroidImg = [fix((xLImg+xRImg)/2),fix((yLImg+yRImg)/2)];

end

%CONVERT ROI COORDINATES TO IMG COORDINATES (VERTICAL)
function [rTopImg, rBottomImg, rCentroidImg] = convertCoordinatesVertical(rTopROI,rBottomROI,rCentroid,roiHalfwidth,roiHalfheight)
%This function takes in the dot positions in the ROI frame of reference
%and outputs coordinates in the origional image frame of reference, all in
%vectorize format [x,y].  Note that x = column and y = row.

%Convert y (row) coordinates 
yTImg = rCentroid(2) - roiHalfheight + rTopROI(2);
yBImg = rCentroid(2) - roiHalfheight + rBottomROI(2);
%Convert x (col) coordinates
xTImg = rCentroid(1) - roiHalfwidth + rTopROI(1);
xBImg = rCentroid(1) - roiHalfwidth + rBottomROI(1);
%Put results into vector format
rTopImg    = [ xTImg, yTImg ];
rBottomImg = [ xBImg, yBImg ];
%Calculate ROI cenntroid as average of two dot coordinates
rCentroidImg = [fix((xTImg+xBImg)/2),fix((yTImg+yBImg)/2)];

end

%CENTROID METHOD DOT LOCATION (HORIZONTAL)
function [rLeft,rRight,rCentroid] = centroidMethodHorizontal(roi,roiHalfwidth,roiHalfheight)
%Function returns the position of the dots rCentroid as well as the
%centroid of the overall image rCentroid
%Calculated by using centroid method, assuming the dots are arranged
%horizontally

%Divide the image in half vertically (left and right)
roiLeft  = roi( : , 1            : roiHalfwidth);
roiRight = roi( : , roiHalfwidth : end         );

%Calculate the x coordinates of the centroids
xLROI = round(sum((sum(roiLeft ,1) .* (1:size(roiLeft ,2))))/sum(sum(roiLeft )));
xRROI = round(sum((sum(roiRight,1) .* (1:size(roiRight,2))))/sum(sum(roiRight)))+roiHalfwidth;
%Calculate the y coordinates of the centroids
yLROI = round(sum((sum(roiLeft ,2) .* (1:size(roiLeft, 1))'))/sum(sum(roiLeft )));
yRROI = round(sum((sum(roiRight,2) .* (1:size(roiRight,1))'))/sum(sum(roiRight)));
%Put results into vector format
rLeft     = [xLROI, yLROI];
rRight    = [xRROI, yRROI];
%Find ROI cenntroid as the average position of the two centroids
rCentroid = [fix((xLROI+xRROI)/2),fix((yLROI+yRROI)/2)];
end

%CENTROID METHOD DOT LOCATION (VERTICAL)
function [rTop,rBottom,rCentroid] = centroidMethodVertical(roi,roiHalfwidth,roiHalfheight)
%Function returns the position of the dots rCentroid as well as the
%centroid of the overall image rCentroid
%Calculated by using centroid method assuming the dots are arranged
%vertically;

%Divide the image in half horizontally (top and bottom)
roiTop    = roi( 1             : roiHalfheight , : );
roiBottom = roi( roiHalfheight : end           , : );

%Calculate the x coordinates of the centroids
xTROI = round(sum((sum(roiTop   ,1) .* (1:size(roiTop   ,2))))/sum(sum(roiTop )));
xBROI = round(sum((sum(roiBottom,1) .* (1:size(roiBottom,2))))/sum(sum(roiBottom)));

%Calculate the y coordinates of the centroids
yTROI = round(sum((sum(roiTop   ,2) .* (1:size(roiTop   ,1))'))/sum(sum(roiTop )));
yBROI = round(sum((sum(roiBottom,2) .* (1:size(roiBottom,1))'))/sum(sum(roiBottom)))+roiHalfheight;
%Put results into vector format
rTop     = [xTROI, yTROI];
rBottom  = [xBROI, yBROI];
%Find ROI cenntroid as the average position of the two centroids
rCentroid = [fix((xTROI+xBROI)/2),fix((yTROI+yBROI)/2)];
end

%CLUSTERING METHOD DOT LOCATION
function [rTop,rBottom,rCentroid] = clusterMethod(roi,clusteringParameters)
%This function is currently a placeholder, will be used later if/when
%clustering is implemented
end

%IMAGE THRESHOLDING - OTSU'S METHOD
function img = threshold(img)
%This function takes in a grayscale matrix and outputs a thresholded,
%binaray matrix according to Otsus Method.

%Generate histogram of image
counts=zeros(256,1);
[m,n]=size(img);
for i = 1:m*n
    counts(img(i)+1)=counts(img(i)+1)+1;
end
%Callculate variances
p = counts / sum(counts);
sigma_b=zeros(256,1);
%%%%%%%%%%%%%%%%55
%POSSIBLE DIV BY ZERO ERRORS HERE?
%%%%%%%%%%%%%%%%%%%%%%
for t = 1 : 256
    q_L = sum(p(1 : t));
    q_H = sum(p(t + 1 : end));
    miu_L = sum(p(1 : t) .* (1 : t)') / q_L;
    miu_H = sum(p(t + 1 : end) .* (t + 1 : 256)') / q_H;
    sigma_b(t) = q_L * q_H * (miu_L - miu_H)^2;
end
% Desired threshold is the max of sigma_b vector
[~,threshold_otsu] = max(sigma_b(:));
% Threshold image as those points above the threshold value
img=(img>threshold_otsu);
end

%INPUT PARSING
function        [dotConfig, locationMethod, centroidOverrideCommand ,rCentroidManualOverride ,viewOptions,roiHalfwidth, roiHalfheight]...
    =parseInputs(dotConfig, locationMethod, centroidOverrideCommand ,rCentroidManualOverride ,viewOptions,roiHalfwidth, roiHalfheight)
% This function parses inputs and corrects potentially harmful/unstable
% inputs.  
locationMethod            = setToBinary(locationMethod);
centroidOverrideCommand   = setToBinary(centroidOverrideCommand);

if centroidOverrideCommand == 1
    if numel(rCentroidManualOverride)~=2
        rCentroidManualOverride = [540,1020];
    end
    if rCentroidManualOverride(2) > 1080 - roiHalfheight - 1
        rCentroidManualOverride(2) = 1080 - roiHalfheight - 1;
    end
    if rCentroidManualOverride(1) > 2040 - roiHalfwidth - 1
        rCentroidManualOverride(1) = 2040 - roiHalfwidth - 1;
    end
    
    if rCentroidManualOverride(2) < roiHalfheight + 1
        rCentroidManualOverride(2) = roiHalfheight + 1;
    end
    if rCentroidManualOverride(1) < roiHalfwidth + 1
        rCentroidManualOverride(1) = roiHalfwidth + 1;
    end
    
    
end

if numel(viewOptions) > 8
    viewOptions = viewOptions(1:8);
end
if numel(viewOptions) < 8
    viewOptions = [0,0,0,0,0,0,0,0];
end
for i=1:8
    viewOptions(i) = setToBinary(viewOptions(i));
end
rCentroidManualOverride=fix(rCentroidManualOverride);
dotConfig = setToBinary(dotConfig);

end

%ROUND TO BINARY VALUE
function [out] = setToBinary(in)
%takes any numerical input and sets it to either 0 or 1 depending on
%what's closer
out = in;
if out>1
    out=1;
end
if out<0
    out=0;
end
if out >0  && out <1
    out=round(out);
end
end

%GET ROI DIMENSIONS
function [roiHalfwidth,roiHalfheight] = getROIDimensions(dotConfig,roiDims)
%This function sets the ROI Dimensions depending on user input
%(dotConfig).


if numel(roiDims)==4 %Check to make sure ROI dimension vector is right length
    for i = 1 : 4   %Saturation, make sure roi dimension vector elements make sense, if not set them to something more reasonable
       if roiDims(i)>200
           roiDims(i)=200;
       end
       
       if roiDims(i)<20
           roiDims(i)=20;
       end
    end
    
    
    
    if dotConfig == 1 %VERTICAL ARRANGEMENT
        roiHalfwidth = roiDims(1);
        roiHalfheight = roiDims(2);
        
    else
        roiHalfwidth = roiDims(3);
        roiHalfheight = roiDims(4);
    end
end

end

%PARSE DOT LOCATIONS
function [r1ROI,r2ROI,rCentroidROI] = parseDotLocations(dotConfig,r1ROI,r2ROI,rCentroidROI,roiHalfwidth,roiHalfheight)
if dotConfig == 0 %HORIZONTAL DOTS
    if isnan(r1ROI(1))
        r1ROI(1)=fix(roiHalfwidth/2);
    end
    if isnan(r1ROI(2))
        r1ROI(2)=roiHalfheight;
    end
    if isnan(r2ROI(1))
        r2ROI(1)=fix(3*roiHalfheight/2);
    end
    if isnan(r2ROI(2))
        r2ROI(2)=roiHalfheight;
    end
else %VERTICAL DOTS
    if isnan(r1ROI(1))
        r1ROI(1)=roiHalfwidth;
    end
    if isnan(r1ROI(2))
        r1ROI(2)=fix(roiHalfheight/2);
    end
    if isnan(r2ROI(1))
        r2ROI(1)=roiHalfwidth;
    end
    if isnan(r2ROI(2))
        r2ROI(2)=fix(3*roiHalfheight/2);
    end
end

if isnan(rCentroidROI(1))
   rCentroidROI(1)=roiHalfwidth;
end

if isnan(rCentroidROI(2))
    rCentroidROI(2) = roiHalfheight;
end


end

== matlab function UNCCModel/cam3A/MATLAB Function ==
  data: r_cam input; d_cam_com output; r_com input; x_dist output; y_dist output; z_dist output
function [d_cam_com , x_dist, y_dist, z_dist] = distanceToCenterOfMass(r_cam , r_com)
%Function exists to calculate the distance between the camera and the
%center of mass in units of length
%#codegen

x_dist = abs(r_cam(1) - r_com(1));
y_dist = abs(r_cam(2) - r_com(2));
z_dist = abs(r_cam(3) - r_com(3));

d_cam_com = ( x_dist^2 + y_dist^2 + z_dist^2 )^(1/2);

== matlab function UNCCModel/cam2/MATLAB Function ==
  data: r_cam input; d_cam_com output; r_com input; x_dist output; y_dist output; z_dist output
function [d_cam_com , x_dist, y_dist, z_dist] = distanceToCenterOfMass(r_cam , r_com)
%Function exists to calculate the distance between the camera and the
%center of mass in units of length
%#codegen

x_dist = abs(r_cam(1) - r_com(1));
y_dist = abs(r_cam(2) - r_com(2));
z_dist = abs(r_cam(3) - r_com(3));

d_cam_com = ( x_dist^2 + y_dist^2 + z_dist^2 )^(1/2);

== matlab function UNCCModel/cam3B/MATLAB Function ==
  data: r_cam input; d_cam_com output; r_com input; x_dist output; y_dist output; z_dist output
function [d_cam_com , x_dist, y_dist, z_dist] = distanceToCenterOfMass(r_cam , r_com)
%Function exists to calculate the distance between the camera and the
%center of mass in units of length
%#codegen

x_dist = abs(r_cam(1) - r_com(1));
y_dist = abs(r_cam(2) - r_com(2));
z_dist = abs(r_cam(3) - r_com(3));

d_cam_com = ( x_dist^2 + y_dist^2 + z_dist^2 )^(1/2);
